simulink model "induction_motor"  (R2019b)
settings: Solver=VariableStepAuto  StartTime=0.0  StopTime=10.0  RelTol=1e-3
values from neighbouring files (symbols this model uses):
  frequency = 0:0.76:76    [main.m]
  slip = fliplr(slip)    [main.m]
  stator_voltage = 0:0.76:76    [main.m]
settings Model: Creator=jamil  LastModifiedBy=jamil

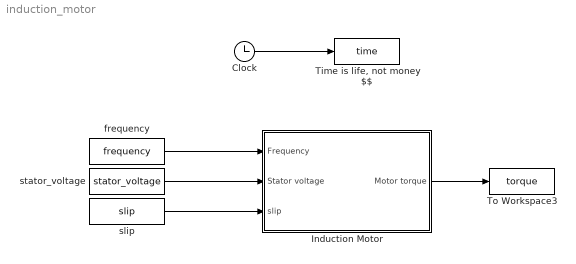
== system induction_motor ==
  Clock : Clock
  Induction Motor : Subsystem
      mask Display: image('induction_motor_pic.jpg'); % Use "Edit Image" on toolstrip to change.
  "Time is life, not money $$" : ToWorkspace  VariableName=time  SampleTime=-1
  To Workspace3 : ToWorkspace  VariableName=torque  SampleTime=-1
  frequency : Constant  Value=frequency
  "slip " : Constant  Value=slip
  "stator_voltage " : Constant  Value=stator_voltage
  wires:
  Clock/1 -> "Time is life, not money $$"/1
  Induction Motor/1(Motor torque) -> To Workspace3/1
  frequency/1 -> Induction Motor/1("Frequency ")
  "stator_voltage "/1 -> Induction Motor/2("Stator voltage ")
  "slip "/1 -> Induction Motor/3("slip ")

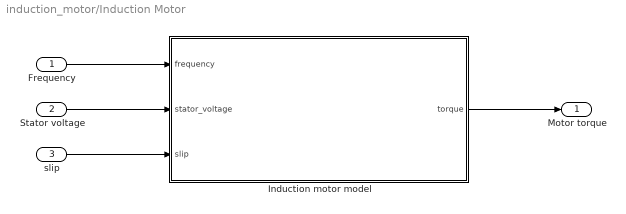
== system induction_motor/Induction Motor ==
  "Frequency " : Inport
  "Stator voltage " : Inport  Port=2
  "slip " : Inport  Port=3
  "Induction motor model " : MATLAB Function  TreatAsAtomicUnit=on
  Motor torque : Outport
  wires:
  "Frequency "/1 -> "Induction motor model "/1(frequency)
  "Induction motor model "/1(torque) -> Motor torque/1
  "Stator voltage "/1 -> "Induction motor model "/2(stator_voltage)
  "slip "/1 -> "Induction motor model "/3(slip)

== matlab function induction_motor/Induction Motor/Induction motor model  ==
  data: frequency input; torque output; stator_voltage input; slip input
function torque = fcn(frequency, stator_voltage, slip)
    % Constant specs
    stator_resistance = 8.56*1e-3;
    stator_leakage_inductance = 0.06292 * 1e-3;
    mutual_inductance = 1.0122 * 1e-3;
    rotor_resistance = 10.20 *1e-3;
    rotor_leakage_inductance = 0.06709 * 1e-3;
    % Variable specs 
    stator_reactance = stator_leakage_inductance * 2 * pi * frequency * 1i;
    rotor_reactance = rotor_leakage_inductance * 2 * pi * frequency * 1i;
    mutual_reactance = mutual_inductance * 2 * pi * frequency * 1i;
    stator_impedance = stator_resistance + stator_reactance;
    rotor_impedance = rotor_resistance + rotor_reactance;
    
     % Descriptive Equations
      equivalent_impedance = stator_impedance + (mutual_reactance.*(((slip -1)./slip).*rotor_resistance+rotor_impedance))./(mutual_reactance+(((slip -1)./slip).*rotor_resistance+rotor_impedance));
      stator_current = stator_voltage ./ equivalent_impedance;
%      % Calculus of torque
     rotor_current = stator_current - (stator_voltage-stator_current.*stator_impedance)./(mutual_reactance);
     mechanical_power = 3 * rotor_current.^2 .* rotor_resistance.*((slip - 1)./slip);
     torque = mechanical_power./(2*pi*frequency);
end
